simulink model "StairCaseWaveGenerator"  (R2020b)
settings: Solver=VariableStepAuto  StartTime=0.0  StopTime=1  FixedStep=1  MaxStep=0.01  RelTol=1e-3
settings Model: Creator=99003778  LastModifiedBy=99003778

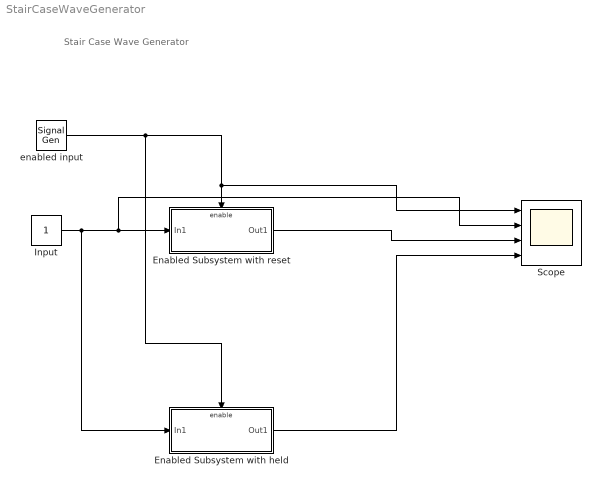
== system StairCaseWaveGenerator ==
  note: Stair Case Wave Generator
  Enabled Subsystem with held : Subsystem  TreatAsAtomicUnit=on
  Enabled Subsystem with reset : Subsystem  TreatAsAtomicUnit=on
  Input : Constant
  Scope : Scope  NumInputPorts=4
  enabled input : SignalGenerator  WaveForm=square  Frequency=3
  wires:
  Input/1 -> Enabled Subsystem with held/1(In1), Scope/2, Enabled Subsystem with reset/1(In1)
  Enabled Subsystem with reset/1(Out1) -> Scope/3
  enabled input/1 -> Enabled Subsystem with held/Enable, Scope/1, Enabled Subsystem with reset/Enable
  Enabled Subsystem with held/1(Out1) -> Scope/4

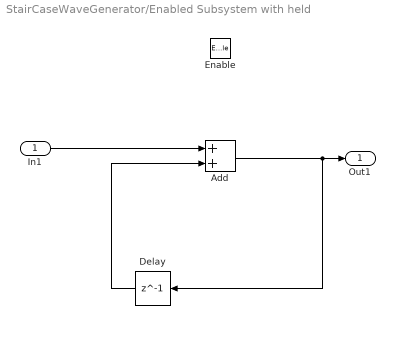
== system StairCaseWaveGenerator/Enabled Subsystem with held ==
  In1 : Inport
  Enable : EnablePort
  Add : Sum
  Delay : Delay  DelayLength=1  InitialCondition=0
  Out1 : Outport
  wires:
  Delay/1 -> Add/2
  In1/1 -> Add/1
  Add/1 -> Out1/1, Delay/1

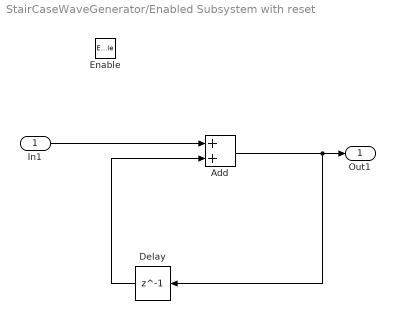
== system StairCaseWaveGenerator/Enabled Subsystem with reset ==
  In1 : Inport
  Enable : EnablePort  StatesWhenEnabling=reset
  Add : Sum
  Delay : Delay  DelayLength=1  InitialCondition=0
  Out1 : Outport
  wires:
  Delay/1 -> Add/2
  In1/1 -> Add/1
  Add/1 -> Out1/1, Delay/1
